simulink model "ZedBoardTest_interface"  (R2014b)
settings: Solver=FixedStepDiscrete  StartTime=0.0  StopTime=inf  RelTol=1e-3
InitFcn:
  | Ts = 1e-3;
undefined symbols (not defined in the file): AXI4, Lite
libraries: axiinterfacelib x6
settings Model: SimulationMode=external  Creator=wchen  LastModifiedBy=dlwalter
settings SolverCC: PositivePriorityOrder=on
settings DataIOCC: SaveOutput=off  SaveTime=off
settings OptimizationCC: OptimizeModelRefInitCode=on  LifeSpan=1  MaxStackSize=64
settings DebuggingCC: UnderspecifiedInitializationDetection=Classic  MergeDetectMultiDrivingBlocksExec=none
settings HardwareCC: ProdLargestAtomicInteger=Long  ProdLargestAtomicFloat=Double  ProdEndianess=LittleEndian  ProdHWDeviceType=ARM Compatible->ARM Cortex  TargetLargestAtomicInteger=Long  TargetLargestAtomicFloat=Double  TargetIntDivRoundTo=Zero  TargetEndianess=LittleEndian  TargetHWDeviceType=ARMCortex  ProdEqTarget=off
settings RTWCC: SystemTargetFile=ert.tlc  TLCOptions=-aInlineSetEventsForThisBaseRateFcn=TLC_FALSE -aSuppressMultiTaskScheduler=TLC_FALSE  TemplateMakefile=ert_default_tmf  Description=Embedded Coder  ProcessScript=idelink_ert_make_rtw_hook  Toolchain=Xilinx ISE Design Suite 14.4
settings CodeAppCC: IgnoreCustomStorageClasses=off
settings ERTTargetCC: ParMdlRefBuildCompliant=off  GeneratePreprocessorConditionals=Disable all  CPPClassGenCompliant=off

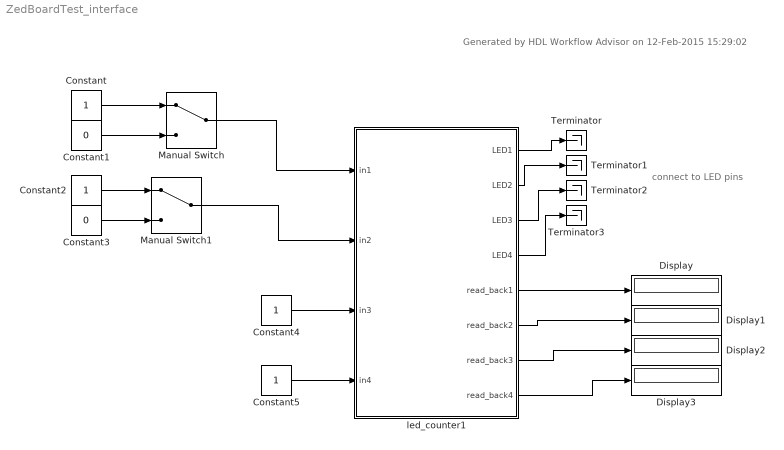
== system ZedBoardTest_interface ==
  note: connect to
      | LED pins
  note: Generated by HDL Workflow Advisor on 12-Feb-2015 15:29:02
  Constant{,2,4..5} (4 alike) : Constant  OutDataTypeStr=boolean  SampleTime=Ts
  Constant1 : Constant  Value=0  OutDataTypeStr=boolean  SampleTime=Ts
  Constant3 : Constant  Value=0  OutDataTypeStr=boolean  SampleTime=Ts
  Display{,1..3} (4 alike) : Display
  Manual Switch : ManualSwitch
  Manual Switch1 : ManualSwitch
  Terminator{,1..3} (4 alike) : Terminator
  led_counter1 : Subsystem  TreatAsAtomicUnit=on  SystemSampleTime=0.001  mask(AXI4-Lite/AXI4 Interface){}
      mask help:
      | This is an automatically generated subsystem block.
      | This contains the AXI4-Lite/AXI4 interface which communicates with the zedboardtest_led_counter_pcore IPCore generated from ZedBoardTest/led_counter subsystem.
      mask Display: disp(sprintf('Xilinx Zynq \nAXI4-Lite/AXI4 Interface'));
  wires:
  led_counter1/8(read_back4) -> Display3/1
  led_counter1/7(read_back3) -> Display2/1
  led_counter1/6(read_back2) -> Display1/1
  led_counter1/4(LED4) -> Terminator3/1
  led_counter1/3(LED3) -> Terminator2/1
  led_counter1/2(LED2) -> Terminator1/1
  led_counter1/1(LED1) -> Terminator/1
  Manual Switch1/1 -> led_counter1/2(in2)
  Constant3/1 -> Manual Switch1/2
  Constant2/1 -> Manual Switch1/1
  Manual Switch/1 -> led_counter1/1(in1)
  Constant1/1 -> Manual Switch/2
  Constant/1 -> Manual Switch/1
  led_counter1/5(read_back1) -> Display/1
  Constant4/1 -> led_counter1/3(in3)
  Constant5/1 -> led_counter1/4(in4)

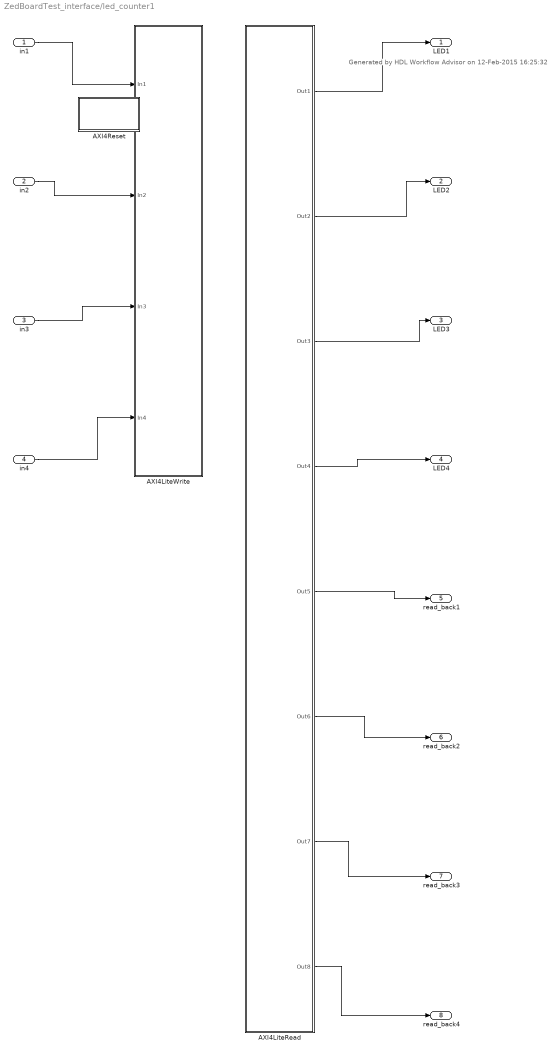
== system ZedBoardTest_interface/led_counter1 ==
  note: Generated by HDL Workflow Advisor on 12-Feb-2015 16:25:32
  in1 : Inport  OutDataTypeStr=boolean
  in2 : Inport  Port=2  OutDataTypeStr=boolean
  in3 : Inport  Port=3  OutDataTypeStr=boolean
  in4 : Inport  Port=4  OutDataTypeStr=boolean
  AXI4LiteRead : Subsystem  Priority=10
  AXI4LiteWrite : Subsystem  Priority=1
  AXI4Reset : Subsystem  mask(System Initialize){ShowInLibBrowser=0}
      mask prompts: ShowInLibBrowser "Simulink:masks:CustCodeMaskParam1_MP"
      settings: CopyFcn=cccopyfcn(gcb)  OpenFcn=ccopenfcn('System Initialize Function')
      mask Help: eval('feval(''rtwprivate'',''rtwhelpview'',''rtw_sys_initialize_block'')');
      mask Display: disp('System\nInitialize');
  LED1 : Outport
  LED2 : Outport  Port=2
  LED3 : Outport  Port=3
  LED4 : Outport  Port=4
  read_back1 : Outport  Port=5
  read_back2 : Outport  Port=6
  read_back3 : Outport  Port=7
  read_back4 : Outport  Port=8
  wires:
  in1/1 -> AXI4LiteWrite/1(In1)
  in2/1 -> AXI4LiteWrite/2(In2)
  in3/1 -> AXI4LiteWrite/3(In3)
  in4/1 -> AXI4LiteWrite/4(In4)
  AXI4LiteRead/1(Out1) -> LED1/1
  AXI4LiteRead/2(Out2) -> LED2/1
  AXI4LiteRead/3(Out3) -> LED3/1
  AXI4LiteRead/4(Out4) -> LED4/1
  AXI4LiteRead/5(Out5) -> read_back1/1
  AXI4LiteRead/6(Out6) -> read_back2/1
  AXI4LiteRead/7(Out7) -> read_back3/1
  AXI4LiteRead/8(Out8) -> read_back4/1

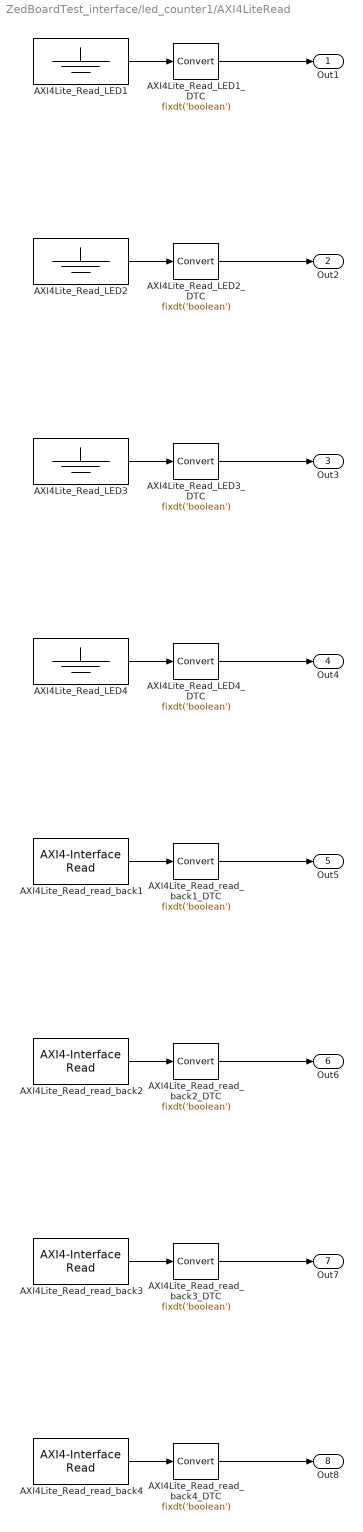
== system ZedBoardTest_interface/led_counter1/AXI4LiteRead ==
  AXI4Lite_Read_LED{1..4} (4 alike) : Ground
  AXI4Lite_Read_LED1_DTC : DataTypeConversion  OutDataTypeStr=fixdt('boolean')  ConvertRealWorld=Stored Integer (SI)
  AXI4Lite_Read_LED2_DTC : DataTypeConversion  OutDataTypeStr=fixdt('boolean')  ConvertRealWorld=Stored Integer (SI)
  AXI4Lite_Read_LED3_DTC : DataTypeConversion  OutDataTypeStr=fixdt('boolean')  ConvertRealWorld=Stored Integer (SI)
  AXI4Lite_Read_LED4_DTC : DataTypeConversion  OutDataTypeStr=fixdt('boolean')  ConvertRealWorld=Stored Integer (SI)
  AXI4Lite_Read_read_back1 : axiinterfacelib/AXI4-Interface Read  Priority=6  AXIInterfaceType=AXI4-Lite  DeviceName=/dev/mwipcore  RegisterOffset=hex2dec('110')  DataType=uint32  DataLength=4096  SampleTime=-1  blockPlatform=ZYNQ  SimulateUsing=Interpreted Execution
  AXI4Lite_Read_read_back1_DTC : DataTypeConversion  OutDataTypeStr=fixdt('boolean')  ConvertRealWorld=Stored Integer (SI)
  AXI4Lite_Read_read_back2 : axiinterfacelib/AXI4-Interface Read  Priority=7  AXIInterfaceType=AXI4-Lite  DeviceName=/dev/mwipcore  RegisterOffset=hex2dec('114')  DataType=uint32  DataLength=4096  SampleTime=-1  blockPlatform=ZYNQ  SimulateUsing=Interpreted Execution
  AXI4Lite_Read_read_back2_DTC : DataTypeConversion  OutDataTypeStr=fixdt('boolean')  ConvertRealWorld=Stored Integer (SI)
  AXI4Lite_Read_read_back3 : axiinterfacelib/AXI4-Interface Read  Priority=8  AXIInterfaceType=AXI4-Lite  DeviceName=/dev/mwipcore  RegisterOffset=hex2dec('118')  DataType=uint32  DataLength=4096  SampleTime=-1  blockPlatform=ZYNQ  SimulateUsing=Interpreted Execution
  AXI4Lite_Read_read_back3_DTC : DataTypeConversion  OutDataTypeStr=fixdt('boolean')  ConvertRealWorld=Stored Integer (SI)
  AXI4Lite_Read_read_back4 : axiinterfacelib/AXI4-Interface Read  Priority=9  AXIInterfaceType=AXI4-Lite  DeviceName=/dev/mwipcore  RegisterOffset=hex2dec('11C')  DataType=uint32  DataLength=4096  SampleTime=-1  blockPlatform=ZYNQ  SimulateUsing=Interpreted Execution
  AXI4Lite_Read_read_back4_DTC : DataTypeConversion  OutDataTypeStr=fixdt('boolean')  ConvertRealWorld=Stored Integer (SI)
  Out1 : Outport
  Out2 : Outport  Port=2
  Out3 : Outport  Port=3
  Out4 : Outport  Port=4
  Out5 : Outport  Port=5
  Out6 : Outport  Port=6
  Out7 : Outport  Port=7
  Out8 : Outport  Port=8
  wires:
  AXI4Lite_Read_read_back2/1 -> AXI4Lite_Read_read_back2_DTC/1
  AXI4Lite_Read_read_back2_DTC/1 -> Out6/1
  AXI4Lite_Read_read_back1_DTC/1 -> Out5/1
  AXI4Lite_Read_read_back1/1 -> AXI4Lite_Read_read_back1_DTC/1
  AXI4Lite_Read_read_back3_DTC/1 -> Out7/1
  AXI4Lite_Read_read_back3/1 -> AXI4Lite_Read_read_back3_DTC/1
  AXI4Lite_Read_read_back4/1 -> AXI4Lite_Read_read_back4_DTC/1
  AXI4Lite_Read_read_back4_DTC/1 -> Out8/1
  AXI4Lite_Read_LED1/1 -> AXI4Lite_Read_LED1_DTC/1
  AXI4Lite_Read_LED1_DTC/1 -> Out1/1
  AXI4Lite_Read_LED3/1 -> AXI4Lite_Read_LED3_DTC/1
  AXI4Lite_Read_LED3_DTC/1 -> Out3/1
  AXI4Lite_Read_LED4/1 -> AXI4Lite_Read_LED4_DTC/1
  AXI4Lite_Read_LED4_DTC/1 -> Out4/1
  AXI4Lite_Read_LED2/1 -> AXI4Lite_Read_LED2_DTC/1
  AXI4Lite_Read_LED2_DTC/1 -> Out2/1

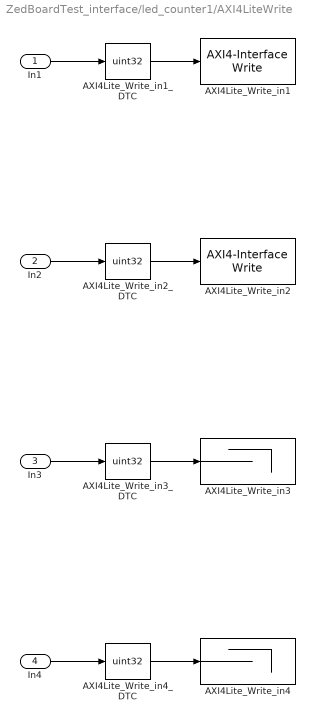
== system ZedBoardTest_interface/led_counter1/AXI4LiteWrite ==
  In1 : Inport
  In2 : Inport  Port=2
  In3 : Inport  Port=3
  In4 : Inport  Port=4
  AXI4Lite_Write_in1 : axiinterfacelib/AXI4-Interface Write  Priority=1  AXIInterfaceType=AXI4-Lite  DeviceName=/dev/mwipcore  RegisterOffset=hex2dec('100')  blockPlatform=ZYNQ  SimulateUsing=Interpreted execution
  AXI4Lite_Write_in1_DTC : DataTypeConversion  OutDataTypeStr=uint32  ConvertRealWorld=Stored Integer (SI)
  AXI4Lite_Write_in2 : axiinterfacelib/AXI4-Interface Write  Priority=2  AXIInterfaceType=AXI4-Lite  DeviceName=/dev/mwipcore  RegisterOffset=hex2dec('104')  blockPlatform=ZYNQ  SimulateUsing=Interpreted execution
  AXI4Lite_Write_in2_DTC : DataTypeConversion  OutDataTypeStr=uint32  ConvertRealWorld=Stored Integer (SI)
  AXI4Lite_Write_in3 : Terminator
  AXI4Lite_Write_in3_DTC : DataTypeConversion  OutDataTypeStr=uint32  ConvertRealWorld=Stored Integer (SI)
  AXI4Lite_Write_in4 : Terminator
  AXI4Lite_Write_in4_DTC : DataTypeConversion  OutDataTypeStr=uint32  ConvertRealWorld=Stored Integer (SI)
  wires:
  In1/1 -> AXI4Lite_Write_in1_DTC/1
  AXI4Lite_Write_in1_DTC/1 -> AXI4Lite_Write_in1/1
  In2/1 -> AXI4Lite_Write_in2_DTC/1
  AXI4Lite_Write_in3_DTC/1 -> AXI4Lite_Write_in3/1
  AXI4Lite_Write_in2_DTC/1 -> AXI4Lite_Write_in2/1
  In3/1 -> AXI4Lite_Write_in3_DTC/1
  In4/1 -> AXI4Lite_Write_in4_DTC/1
  AXI4Lite_Write_in4_DTC/1 -> AXI4Lite_Write_in4/1

== system ZedBoardTest_interface/led_counter1/AXI4Reset ==
